simulink model "px4demo_tune"  (R2014b)
settings: Solver=FixedStepDiscrete  SolverMode=SingleTasking  StartTime=0.0  StopTime=200  RelTol=1e-3
undefined symbols (not defined in the file): PX4_TUNE_ENUM
libraries: simulink x1, pixhawk_sllib x1
settings Model: Creator=skuznick  LastModifiedBy=skuznick
settings OptimizationCC: InlineParams=on  OptimizeModelRefInitCode=on  LifeSpan=1  MaxStackSize=64
settings HardwareCC: ProdLargestAtomicInteger=Long  ProdLargestAtomicFloat=Double  ProdEndianess=LittleEndian  ProdHWDeviceType=ARM Compatible->ARM Cortex
settings RTWCC: SystemTargetFile=ert.tlc  TLCOptions=-aInlineSetEventsForThisBaseRateFcn=TLC_FALSE -aSuppressMultiTaskScheduler=TLC_FALSE  TemplateMakefile=ert_default_tmf  Description=Embedded Coder  GenerateReport=on  ProcessScript=ert_make_rtw_hook  Toolchain=Pixhawk Toolchain  IncludeHyperlinkInReport=on  LaunchReport=on  GenerateTraceReport=on  GenerateTraceReportSl=on  GenerateTraceReportSf=on  GenerateTraceReportEml=on  GenerateCodeMetricsReport=on
settings CodeAppCC: IgnoreCustomStorageClasses=off

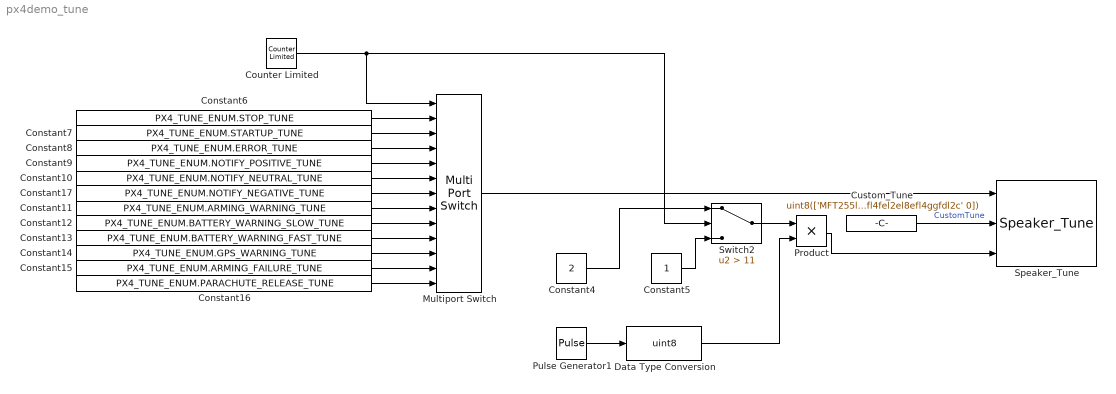
== system px4demo_tune ==
  Constant10 : Constant  Value=PX4_TUNE_ENUM.NOTIFY_NEUTRAL_TUNE  OutDataTypeStr=Enum: PX4_TUNE_ENUM
  Constant11 : Constant  Value=PX4_TUNE_ENUM.ARMING_WARNING_TUNE  OutDataTypeStr=Enum: PX4_TUNE_ENUM
  Constant12 : Constant  Value=PX4_TUNE_ENUM.BATTERY_WARNING_SLOW_TUNE  OutDataTypeStr=Enum: PX4_TUNE_ENUM
  Constant13 : Constant  Value=PX4_TUNE_ENUM.BATTERY_WARNING_FAST_TUNE  OutDataTypeStr=Enum: PX4_TUNE_ENUM
  Constant14 : Constant  Value=PX4_TUNE_ENUM.GPS_WARNING_TUNE  OutDataTypeStr=Enum: PX4_TUNE_ENUM
  Constant15 : Constant  Value=PX4_TUNE_ENUM.ARMING_FAILURE_TUNE  OutDataTypeStr=Enum: PX4_TUNE_ENUM
  Constant16 : Constant  Value=PX4_TUNE_ENUM.PARACHUTE_RELEASE_TUNE  OutDataTypeStr=Enum: PX4_TUNE_ENUM
  Constant17 : Constant  Value=PX4_TUNE_ENUM.NOTIFY_NEGATIVE_TUNE  OutDataTypeStr=Enum: PX4_TUNE_ENUM
  Constant4 : Constant  Value=2  OutDataTypeStr=uint8
  Constant5 : Constant  OutDataTypeStr=uint8
  Constant6 : Constant  Value=PX4_TUNE_ENUM.STOP_TUNE  OutDataTypeStr=Enum: PX4_TUNE_ENUM
  Constant7 : Constant  Value=PX4_TUNE_ENUM.STARTUP_TUNE  OutDataTypeStr=Enum: PX4_TUNE_ENUM
  Constant8 : Constant  Value=PX4_TUNE_ENUM.ERROR_TUNE  OutDataTypeStr=Enum: PX4_TUNE_ENUM
  Constant9 : Constant  Value=PX4_TUNE_ENUM.NOTIFY_POSITIVE_TUNE  OutDataTypeStr=Enum: PX4_TUNE_ENUM
  Counter Limited : simulink/Sources/Counter Limited  uplimit=12  tsamp=10
  Custom_Tune : Constant  Value=uint8(['MFT255l4o2eel2el4eel2el4egl3cl8dl1el4ffl3fl8fl4fel2el8eel4eddel2dgl4eel2el4eel2el4egl3cl8dl1el4ffl3fl8fl4fel2el8efl4ggfdl2c' 0])  OutDataTypeStr=uint8
  Data Type Conversion : DataTypeConversion  OutDataTypeStr=uint8
  Multiport Switch : MultiPortSwitch  DataPortOrder=Zero-based contiguous  Inputs=12  DiagnosticForDefault=None
  Product : Product  OutDataTypeStr=Inherit: Same as first input
  Pulse Generator1 : DiscretePulseGenerator  PulseType=Time based  Period=10  PulseWidth=50
  Speaker_Tune : pixhawk_sllib/Speaker_Tune
  Switch2 : Switch  Criteria=u2 > Threshold  Threshold=11
  wires:
  Pulse Generator1/1 -> Data Type Conversion/1
  Constant7/1 -> Multiport Switch/3
  Constant9/1 -> Multiport Switch/5
  Constant8/1 -> Multiport Switch/4
  Constant10/1 -> Multiport Switch/6
  Constant13/1 -> Multiport Switch/10
  Constant15/1 -> Multiport Switch/12
  Constant14/1 -> Multiport Switch/11
  Constant12/1 -> Multiport Switch/9
  Constant6/1 -> Multiport Switch/2
  Constant11/1 -> Multiport Switch/8
  Constant17/1 -> Multiport Switch/7
  Constant16/1 -> Multiport Switch/13
  Multiport Switch/1 -> Speaker_Tune/1
  Custom_Tune/1 -> Speaker_Tune/2  "CustomTune"
  Data Type Conversion/1 -> Product/2
  Product/1 -> Speaker_Tune/3
  Counter Limited/1 -> Switch2/2, Multiport Switch/1
  Constant4/1 -> Switch2/1
  Constant5/1 -> Switch2/3
  Switch2/1 -> Product/1
